simulink model "HANcoder_E407_GTSync_v3"  (R2018b)
settings: Solver=FixedStepDiscrete  StartTime=0.0  StopTime=1  FixedStep=0.01  RelTol=1e-3
PreLoadFcn:
  | librarySetup
  | eval([bdroot,'_startup']) %Calling [modelName]_startup.m
values from neighbouring files (symbols this model uses):
  frequency_IRQ = 100    [HANcoder_E407_GTSync_startup.m]    (also in HANcoder_E407_GTSync_v3_clean_startup.m = 99; HANcoder_E407_GTSync_v3_startup.m = 99)
  HANtuneOverride = Simulink.Parameter    [HANcoder_E407_GTSync_startup.m]    (also in HANcoder_E407_GTSync_v3_clean_startup.m; HANcoder_E407_GTSync_v3_startup.m)
  LED_ticks_toggle = 10000    [HANcoder_E407_GTSync_startup.m]    (also in HANcoder_E407_GTSync_v3_clean_startup.m; HANcoder_E407_GTSync_v3_startup.m)
  Master_Role = 1    [HANcoder_E407_GTSync_v3_clean_startup.m]    (also in HANcoder_E407_GTSync_v3_startup.m)
  matrix_rows = 2    [HANcoder_E407_GTSync_v3_clean_startup.m]    (also in HANcoder_E407_GTSync_v3_startup.m)
  Sync_ID = 1    [HANcoder_E407_GTSync_v3_clean_startup.m]    (also in HANcoder_E407_GTSync_v3_startup.m)
  time_difference_threshold = 500    [HANcoder_E407_GTSync_v3_clean_startup.m]    (also in HANcoder_E407_GTSync_v3_startup.m = 100)
  TM0 = 100    [HANcoder_E407_GTSync_v3_clean_startup.m]    (also in HANcoder_E407_GTSync_v3_startup.m = 0)
  TM1 = 20000    [HANcoder_E407_GTSync_v3_clean_startup.m]    (also in HANcoder_E407_GTSync_v3_startup.m = 25000)
  TM2 = 30000    [HANcoder_E407_GTSync_v3_clean_startup.m]    (also in HANcoder_E407_GTSync_v3_startup.m = 37500)
  TM3 = 40000    [HANcoder_E407_GTSync_v3_clean_startup.m]    (also in HANcoder_E407_GTSync_v3_startup.m)
  Vote1_ID = 12    [HANcoder_E407_GTSync_v3_clean_startup.m]    (also in HANcoder_E407_GTSync_v3_startup.m)
  Vote2_ID = 22    [HANcoder_E407_GTSync_v3_clean_startup.m]    (also in HANcoder_E407_GTSync_v3_startup.m)
  Vote3_ID = 32    [HANcoder_E407_GTSync_v3_clean_startup.m]    (also in HANcoder_E407_GTSync_v3_startup.m)
undefined symbols (not defined in the file or in its folder): votes
libraries: HANcoder_STM32_Target x20, simulink x3, simulink_extras x1
(part 1 of 2)
CloseFcn:
  | rtwprivate ssgencode ModelCloseRequest mytest
settings Model: Creator=Jason van Kolfschoten  LastModifiedBy=jordy
settings SolverCC: PositivePriorityOrder=on
settings DataIOCC: LimitDataPoints=on  SaveFormat=Array  SignalLoggingSaveFormat=ModelDataLogs  SaveOutput=off  SaveTime=off
settings OptimizationCC: BlockReduction=off  DefaultParameterBehavior=Inlined  InlineInvariantSignals=on  ExpressionDepthLimit=2147483647  StateBitsets=on  DataBitsets=on  ZeroExternalMemoryAtStartup=off  ZeroInternalMemoryAtStartup=off  InitFltsAndDblsToZero=on  NoFixptDivByZeroProtection=on  EfficientFloat2IntCast=on  LifeSpan=inf
settings DebuggingCC: SaveWithDisabledLinksMsg=none  SaveWithParameterizedLinksMsg=none  CheckSSInitialOutputMsg=off  UnderspecifiedInitializationDetection=Classic  MergeDetectMultiDrivingBlocksExec=none  SignalResolutionControl=TryResolveAll  SolverPrmCheckMsg=warning  InheritedTsInSrcMsg=none  MultiTaskDSMMsg=warning  MultiTaskCondExecSysMsg=none  ParameterPrecisionLossMsg=none  FcnCallInpInsideContextMsg=warning  StateNameClashWarn=warning  SFUnexpectedBacktrackingDiag=warning  SFNoUnconditionalDefaultTransitionDiag=warning  SFExecutionAtInitializationDiag=none
settings HardwareCC: ProdBitPerPointer=32  ProdBitPerSizeT=32  ProdBitPerPtrDiffT=32  ProdLargestAtomicFloat=None  ProdIntDivRoundTo=Undefined  ProdWordSize=32  ProdHWDeviceType=Generic->32-bit Embedded Processor  TargetEndianess=LittleEndian  TargetHWDeviceType=Infineon->TriCore
settings ModelReferenceCC: PropagateSignalLabelsOutOfModel=off
settings SFSimCC: SimUseLocalCustomCode=off  MATLABDynamicMemAlloc=off
settings RTWCC: SystemTargetFile=ert.tlc  MakeCommand=make_rtw SHELL= HANcoder_PORTABLE=1 HANcoder_BOOTLOADER=1  TemplateMakefile=STM32_E407_gcc.tmf  Description=Real-Time Workshop Embedded Coder (no auto configuration)  RTWUseLocalCustomCode=off
settings CodeAppCC: ForceParamTrailComments=on  IgnoreCustomStorageClasses=off  SimulinkDataObjDesc=on  CustomSymbolStrGlobalVar=rt$N$M  CustomSymbolStrType=$N$M  CustomSymbolStrFcn=$N$M$F  CustomSymbolStrMacro=$N$M  InsertBlockDesc=on  StateflowObjectComments=on  InternalIdentifier=Classic
settings ERTTargetCC: TargetFcnLib=ansi_tfl_tmw.mat  MultiwordLength=2048  IncludeMdlTerminateFcn=off  SuppressErrorStatus=on  SupportNonFinite=off  GenerateASAP2=on  InlinedParameterPlacement=NonHierarchical  ERTCustomFileTemplate=example_file_process.tlc  ConvertIfToSwitch=off  SuppressUnreachableDefaultCases=off
settings ConfigComp: CovMetricSettings=dw  CovHtmlReporting=on  CovSaveCumulativeToWorkspaceVar=on  CovSaveSingleToWorkspaceVar=on  CovExternalEMLEnable=off  DVMaxProcessTime=600  DVDisplayUnsatisfiableObjectives=on  DVAutomaticStubbing=off  DVModelCoverageObjectives=MCDC  DVMaxTestCaseSteps=500  DVTestSuiteOptimization=CombinedObjectives  DVDetectActiveLogic=on  DVSaveHarnessModel=on

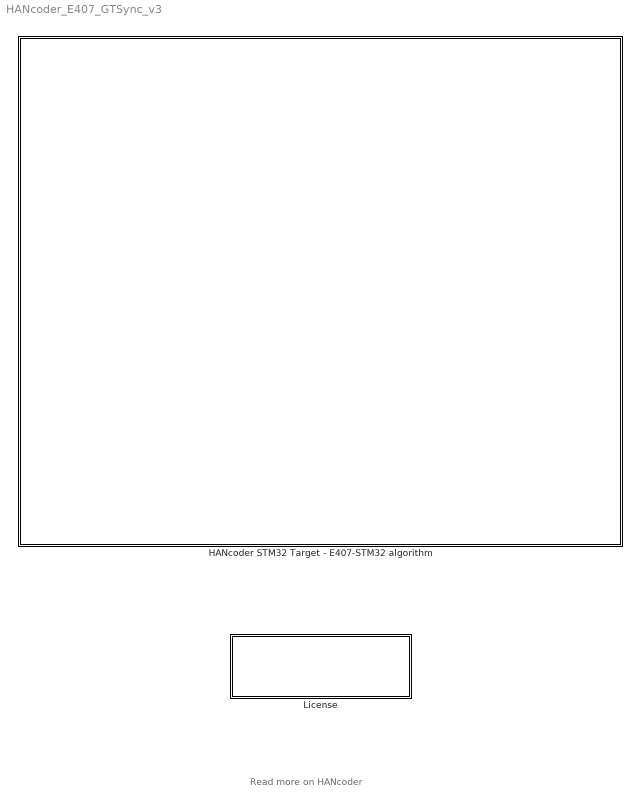
== system HANcoder_E407_GTSync_v3 ==
  note: Read more on HANcoder
  HANcoder STM32 Target - E407-STM32 algorithm : Subsystem  mask(TopLevelSubsystem){}
      settings: CopyFcn=HANcoderChecks('Copy');  NameChangeFcn=HANcoderChecks('NameChangeE407');  MoveFcn=HANcoderChecks('MoveE407');
      mask Display: image(imread('STM32_E407_HAN.jpg'))
  License : Subsystem  mask(License){}
      settings: NameChangeFcn=HANcoderChecks('NameChangeLicenseBlock');  OpenFcn=winopen('License.pdf')  MoveFcn=HANcoderChecks('MoveLicenseBlock');
      mask Display: disp(['End-User License Agreement\n','please read before use']);

== system HANcoder_E407_GTSync_v3/HANcoder STM32 Target - E407-STM32 algorithm ==
  note: Template model
  note: Global Variables
  Algorithm : Subsystem
  Base Sample Time config : HANcoder_STM32_Target/STM32-E407/System Config/Base Sample Time config  Tag=HANcoder_TARGET_STM32_E407  Description=HANcoder Target STM32-E407 blockset version 0.5  baseSampleTime=10  extraStack=0
      settings: SourceProductName=HANcoder STM32 Target
  Build settings : HANcoder_STM32_Target/STM32-E407/System Config/Build settings  Tag=HANcoder_TARGET_STM32_E407  AutoASAP2add=on  AutoFlash=USB
      settings: SourceProductName=HANcoder STM32 Target
  CAN config : HANcoder_STM32_Target/STM32-E407/System Config/CAN config  Tag=HANcoder_TARGET_STM32_E407  txBufSize=64  evBufSize=8  canBus1=off  baudRate1=500  rxMask1=hex2dec('00000000')  rxCode1=hex2dec('00000000')  rxMode1=Receive only 11-bit message identifiers  canBus2=on  baudRate2=500  rxMask2=hex2dec('00000000')  rxCode2=hex2dec('00000000')  rxMode2=Receive only 11-bit message identifiers
      settings: SourceProductName=HANcoder STM32 Target
  Custom ID config : HANcoder_STM32_Target/STM32-E407/System Config/Custom ID config  Tag=HANcoder_TARGET_STM32_E407  softID=softwareID  softNUM=1
      settings: SourceProductName=HANcoder STM32 Target
  Data Store Memory2 : DataStoreMemory  DataStoreName=local_ticks_mem_IRQ  ReadBeforeWriteMsg=warning  WriteAfterWriteMsg=warning  WriteAfterReadMsg=warning  ShowAdditionalParam=off  OutDataTypeStr=uint32
  Global Ticks Increment : Subsystem
  Inputs : Subsystem
  Operation Mode : Subsystem
  Outputs : Subsystem
  System information : Subsystem
  XCP on CAN config : HANcoder_STM32_Target/STM32-E407/System Config/XCP on CAN config  Tag=HANcoder_TARGET_STM32_E407  canBus=CAN 2  croID=hex2dec('665')  dtoID=hex2dec('666')
      settings: SourceProductName=HANcoder STM32 Target
  XCP on USB config : HANcoder_STM32_Target/STM32-E407/System Config/XCP on USB config  Tag=HANcoder_TARGET_STM32_E407
      settings: SourceProductName=HANcoder STM32 Target
  wires:
  Operation Mode/1(Clock_State) -> Global Ticks Increment/1(Clock_State)
  Inputs/1(Button) -> Operation Mode/1(Button_State), Algorithm/1(Button)

== system HANcoder_E407_GTSync_v3/License ==

== system HANcoder_E407_GTSync_v3/HANcoder STM32 Target - E407-STM32 algorithm/Algorithm ==
  note: The button or the HANtuneOverride parameter
      | switches between the two frequencies.
  note: Here the algorithm can be placed. No hardware dependent blocks should be used here.
  note: Switch LED frequency when button is pressed
  Button : Inport
  10Hz Counter Limiter : simulink/Sources/Counter Limited  uplimit=1  tsamp=0.1
  5Hz Counter Limited : simulink/Sources/Counter Limited  uplimit=1  tsamp=0.2
  Constant : Constant  Value=HANtuneOverride  OutDataTypeStr=boolean
  Data Type Conversion : DataTypeConversion  OutDataTypeStr=boolean
  Logical Operator : Logic  Operator=OR  AllPortsSameDT=off  OutDataTypeStr=boolean
  Switch : Switch  Criteria=u2 > Threshold
  Terminator : Terminator
  wires:
  Data Type Conversion/1 -> Terminator/1  "LedValue"
  5Hz Counter Limited/1 -> Switch/3
  Switch/1 -> Data Type Conversion/1
  Button/1 -> Logical Operator/2
  Logical Operator/1 -> Switch/2
  Constant/1 -> Logical Operator/1
  10Hz Counter Limiter/1 -> Switch/1

== system HANcoder_E407_GTSync_v3/HANcoder STM32 Target - E407-STM32 algorithm/Global Ticks Increment ==
  Clock_State : Inport
  CAN Management : Subsystem
  Compare Event IRQ : HANcoder_STM32_Target/STM32-E407/Timer Outputs/Compare Event IRQ  Tag=HANcoder_TARGET_STM32_E407  pin=TIM4 - CON PD - 15 - 5V Tolerant
      settings: SourceProductName=HANcoder STM32 Target
  Constant1 : Constant  Value=frequency_IRQ - 1  OutDataTypeStr=uint16
  Constant2 : Constant  Value=3  OutDataTypeStr=uint8
  Data Store Memory2 : DataStoreMemory  DataStoreName=message_buffer  ReadBeforeWriteMsg=warning  WriteAfterWriteMsg=warning  WriteAfterReadMsg=warning  ShowAdditionalParam=off  OutDataTypeStr=uint32
  Digital Clock : DigitalClock  SampleTime=0.01
  Function-Call Subsystem : Subsystem  TreatAsAtomicUnit=on
  Output Compare Init1 : Subsystem  Tag=HANcoder_TARGET_STM32_E407  AncestorBlock=HANcoder_STM32_Target/STM32-E407/Timer Outputs/Output Compare Init  mask(Output Compare Init){moduleID=TIM4 - CON PD - 15 & 16 &n/a & n/a, frequency=1000000, enableIRQoutput=off}
      mask prompts: moduleID "Timer module"; frequency "Frequency (free running counter) [Hz]"; enableIRQoutput "Enable IRQ output"
      mask help:
      | Function
      | ========
      | Initializes the timer module to allow output compare functionality on the
      | module's channels.
      |
      | Parameters
      | ==========
      | Timer Module:
      |   Selects the timer module.
      |
      | Frequency:
      |   Frequency at which the 16-bit free running counter counts.
      |
      | Enable IRQ output
      |   Controls whether or not the IRQ output is available.
      |
      | Outport
      | =======
      | IRQ
      |   Allows connection of a function call subsystem for the free running
      |   counter overflow event.
      mask init:
      | moduleIDInfoStr = sfcn_timeout_init_mcb(2, moduleID, frequency, enableIRQoutput);
      settings: CopyFcn=sfcn_timeout_init_chk();  MoveFcn=drawLogos
      mask Help: web('sfcn_timeout_init.html');
      mask TypeOptions moduleID: TIM1 - CON PE - 12 & 14 & 16 & 17 | TIM2 - CON4 - D13 & n/a & n/a & n/a | TIM3 - CON4 - D12 & D11 & n/a & n/a | TIM4 - CON PD - 15 & 16 &n/a & n/a | TIM8 - UEXT - 3 & 4 & n/a & n/a | TIM9 - CON3 - D4 & D5 or PE - 8 & 9 | TIM10 - CON2 - A1 or CON PF - 9 | TIM11 - CON2 - A2 or CON PF - 10 | TIM13 - CON2 - A3 or CON PF - 11 | TIM14 - CON2 - A4 or CON PF - 12
      mask Callback moduleID: sfcn_timeout_init_chk();
      mask Display: fprintf('Output Compare Init\n%s', moduleIDInfoStr);patch([135 141 141],[8 14 2],[1 0 0]);patch([143 143 149],[14 2 8],[0 0 0.35]);
  Schedule Compare Event1 : HANcoder_STM32_Target/STM32-E407/Timer Outputs/Schedule Compare Event  Tag=HANcoder_TARGET_STM32_E407  pin=TIM4 - CON PD - 15 - 5V Tolerant  tsamp=-1
      settings: SourceProductName=HANcoder STM32 Target
  Send : Subsystem
  Terminator : Terminator
  wires:
  Clock_State/1 -> Function-Call Subsystem/1(Clock_State)
  Digital Clock/1 -> Terminator/1  "simulation_time"
  Constant2/1 -> Schedule Compare Event1/2
  Constant1/1 -> Schedule Compare Event1/1
  Compare Event IRQ/1 -> Function-Call Subsystem/Trigger
  CAN Management/1(Send New Msg) -> Send/Trigger
  Function-Call Subsystem/1(activate_CAN_management) -> CAN Management/Trigger

== system HANcoder_E407_GTSync_v3/HANcoder STM32 Target - E407-STM32 algorithm/Inputs ==
  note: The inputs and outputs are kept in a separate subsystem, this way the algorithm can easily be transferred to different hardware
  Digital Input : HANcoder_STM32_Target/STM32-E407/Digital Inputs/Digital Input  Tag=HANcoder_TARGET_STM32_E407  pinID=WKUP button  config=Pulldown  tsamp=-1
      settings: SourceProductName=HANcoder STM32 Target
  Button : Outport
  wires:
  Digital Input/1 -> Button/1

== system HANcoder_E407_GTSync_v3/HANcoder STM32 Target - E407-STM32 algorithm/Operation Mode ==
  note: Operation Mode
      | There are two modes of operation:
      | ( 0 ) Idle (Clock Off)
      | ( 1 ) Counting (Clock On)
      | In order to switch from one to the other the Olimexino button
      | must be pressed once. In this subsystem, with every negative
      | edge of the Button State, the Operation Mode will change from
      | one to the other.
  Button_State : Inport
  Constant : Constant  OutDataTypeStr=boolean
  Flip Flop T : Subsystem
  Clock_State : Outport
  wires:
  Constant/1 -> Flip Flop T/1(T)
  Button_State/1 -> Flip Flop T/2(Clk)
  Flip Flop T/1(Q) -> Clock_State/1

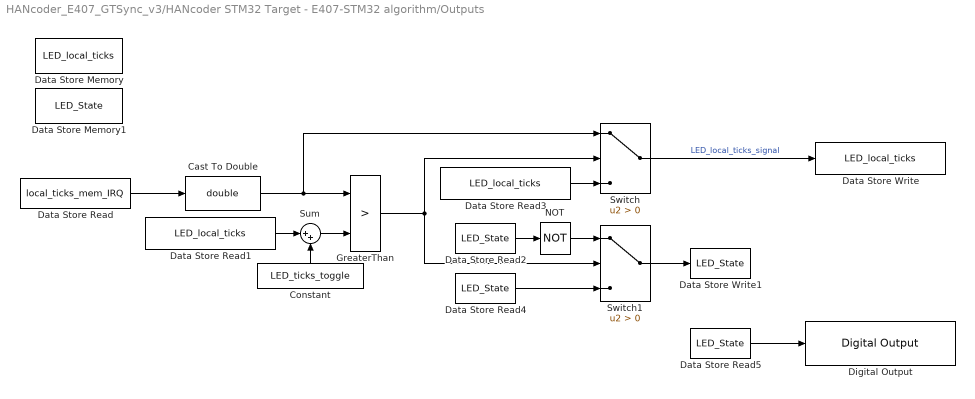
== system HANcoder_E407_GTSync_v3/HANcoder STM32 Target - E407-STM32 algorithm/Outputs ==
  Cast To Double : DataTypeConversion  OutDataTypeStr=double
  Constant : Constant  Value=LED_ticks_toggle
  Data Store Memory : DataStoreMemory  DataStoreName=LED_local_ticks  ReadBeforeWriteMsg=warning  WriteAfterWriteMsg=warning  WriteAfterReadMsg=warning  ShowAdditionalParam=off
  Data Store Memory1 : DataStoreMemory  DataStoreName=LED_State  ReadBeforeWriteMsg=warning  WriteAfterWriteMsg=warning  WriteAfterReadMsg=warning  ShowAdditionalParam=off  OutDataTypeStr=boolean
  Data Store Read : DataStoreRead  DataStoreName=local_ticks_mem_IRQ
  Data Store Read1 : DataStoreRead  DataStoreName=LED_local_ticks
  Data Store Read2 : DataStoreRead  DataStoreName=LED_State
  Data Store Read3 : DataStoreRead  DataStoreName=LED_local_ticks
  Data Store Read4 : DataStoreRead  DataStoreName=LED_State
  Data Store Read5 : DataStoreRead  DataStoreName=LED_State
  Data Store Write : DataStoreWrite  DataStoreName=LED_local_ticks
  Data Store Write1 : DataStoreWrite  DataStoreName=LED_State
  Digital Output : HANcoder_STM32_Target/STM32-E407/Digital Outputs/Digital Output  Tag=HANcoder_TARGET_STM32_E407  pinID=LED  config=Push pull  tsamp=-1
      settings: SourceProductName=HANcoder STM32 Target
  GreaterThan : RelationalOperator  Operator=>  OutDataTypeStr=boolean  RndMeth=Simplest
  NOT : Logic  Operator=NOT  IconShape=distinctive  AllPortsSameDT=off  OutDataTypeStr=boolean
  Sum : Sum  Inputs=|++
  Switch : Switch  Criteria=u2 > Threshold
  Switch1 : Switch  Criteria=u2 > Threshold
  wires:
  Data Store Read1/1 -> Sum/1
  Sum/1 -> GreaterThan/2
  Constant/1 -> Sum/2
  GreaterThan/1 -> Switch/2, Switch1/2
  Switch/1 -> Data Store Write/1  "LED_local_ticks_signal"
  Data Store Read/1 -> Cast To Double/1
  Data Store Read3/1 -> Switch/3
  Cast To Double/1 -> GreaterThan/1, Switch/1
  Switch1/1 -> Data Store Write1/1
  Data Store Read2/1 -> NOT/1
  NOT/1 -> Switch1/1
  Data Store Read4/1 -> Switch1/3
  Data Store Read5/1 -> Digital Output/1

== system HANcoder_E407_GTSync_v3/HANcoder STM32 Target - E407-STM32 algorithm/System information ==
  note: These blocks check the free memory: stack and heap and the CPU load,
      | this way you can see whether your software demands too much of the microcontroller
  Get CPU load : HANcoder_STM32_Target/STM32-E407/System Management/Get CPU load  Tag=HANcoder_TARGET_STM32_E407  mode=Current CPU load  tsamp=-1
      settings: SourceProductName=HANcoder STM32 Target
  Get free Heap : HANcoder_STM32_Target/STM32-E407/System Management/Get free Heap  Tag=HANcoder_TARGET_STM32_E407  tsamp=-1
      settings: SourceProductName=HANcoder STM32 Target
  Get free Stack : HANcoder_STM32_Target/STM32-E407/System Management/Get free Stack  Tag=HANcoder_TARGET_STM32_E407  taskIdx=Application Control Task  tsamp=-1
      settings: SourceProductName=HANcoder STM32 Target
  Terminator : Terminator
  Terminator1 : Terminator
  Terminator2 : Terminator
  wires:
  Get CPU load/1 -> Terminator1/1  "SI_CPUload"
  Get free Stack/1 -> Terminator/1  "SI_FreeStack"
  Get free Heap/1 -> Terminator2/1  "SI_FreeHeap"

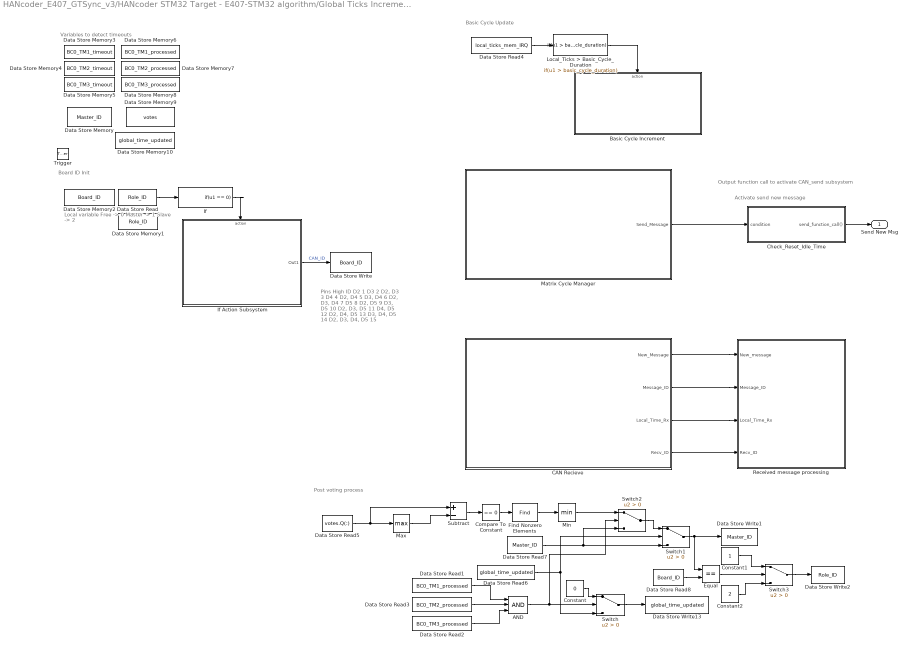
== system HANcoder_E407_GTSync_v3/HANcoder STM32 Target - E407-STM32 algorithm/Global Ticks Increment/CAN Management ==
  note: Post voting process
  note: Variables to detect timeouts
  note: Output function call to activate CAN_send subsystem
  note: Local variable
      |    Free     -> 0
      |    Master -> 1
      |    Slave   -> 2
  note: Pins High      		ID
      | D2                 		1
      | D3				2
      | D2, D3			3
      | D4				4
      | D2, D4			5
      | D3, D4			6
      | D2, D3, D4		7
      | D5				8
      | D2, D5			9
      | D3, D5			10
      | D2, D3, D5		11
      | D4, D5			12
      | D2, D4, D5		13
      | D3, D4, D5		14
      | D2, D3, D4, D5	15
  note: Board ID Init
  note: Activate send new message
  note: Basic Cycle Update
  Trigger : TriggerPort  TriggerType=function-call  VariantControl=Variant  PortDimensions=1
  AND : Logic  Inputs=3  IconShape=distinctive  AllPortsSameDT=off  OutDataTypeStr=boolean
  Basic Cycle Increment : Subsystem  TreatAsAtomicUnit=on
  CAN Recieve : Subsystem
  Check_Reset_Idle_Time : Stateflow chart  TreatAsAtomicUnit=on
  Compare To Constant : simulink/Logic and Bit Operations/Compare To Constant  relop===  const=0  OutDataTypeStr=boolean
  Constant : Constant  Value=0
  Constant1 : Constant
  Constant2 : Constant  Value=2
  Data Store Memory : DataStoreMemory  DataStoreName=Master_ID  ReadBeforeWriteMsg=warning  WriteAfterWriteMsg=warning  WriteAfterReadMsg=warning  InitialValue=1  ShowAdditionalParam=off
  Data Store Memory1 : DataStoreMemory  DataStoreName=Role_ID  ReadBeforeWriteMsg=warning  WriteAfterWriteMsg=warning  WriteAfterReadMsg=warning  ShowAdditionalParam=off
  Data Store Memory10 : DataStoreMemory  DataStoreName=global_time_updated  ReadBeforeWriteMsg=warning  WriteAfterWriteMsg=warning  WriteAfterReadMsg=warning  ShowAdditionalParam=off  OutDataTypeStr=boolean
  Data Store Memory2 : DataStoreMemory  DataStoreName=Board_ID  ReadBeforeWriteMsg=warning  WriteAfterWriteMsg=warning  WriteAfterReadMsg=warning  ShowAdditionalParam=off
  Data Store Memory3 : DataStoreMemory  DataStoreName=BC0_TM1_timeout  ReadBeforeWriteMsg=warning  WriteAfterWriteMsg=warning  WriteAfterReadMsg=warning  ShowAdditionalParam=off  OutDataTypeStr=boolean
  Data Store Memory4 : DataStoreMemory  DataStoreName=BC0_TM2_timeout  ReadBeforeWriteMsg=warning  WriteAfterWriteMsg=warning  WriteAfterReadMsg=warning  ShowAdditionalParam=off  OutDataTypeStr=boolean
  Data Store Memory5 : DataStoreMemory  DataStoreName=BC0_TM3_timeout  ReadBeforeWriteMsg=warning  WriteAfterWriteMsg=warning  WriteAfterReadMsg=warning  ShowAdditionalParam=off  OutDataTypeStr=boolean
  Data Store Memory6 : DataStoreMemory  DataStoreName=BC0_TM1_processed  ReadBeforeWriteMsg=warning  WriteAfterWriteMsg=warning  WriteAfterReadMsg=warning  ShowAdditionalParam=off  OutDataTypeStr=boolean
  Data Store Memory7 : DataStoreMemory  DataStoreName=BC0_TM2_processed  ReadBeforeWriteMsg=warning  WriteAfterWriteMsg=warning  WriteAfterReadMsg=warning  ShowAdditionalParam=off  OutDataTypeStr=boolean
  Data Store Memory8 : DataStoreMemory  DataStoreName=BC0_TM3_processed  ReadBeforeWriteMsg=warning  WriteAfterWriteMsg=warning  WriteAfterReadMsg=warning  ShowAdditionalParam=off  OutDataTypeStr=boolean
  Data Store Memory9 : DataStoreMemory  DataStoreName=votes  ReadBeforeWriteMsg=warning  WriteAfterWriteMsg=warning  WriteAfterReadMsg=warning  ShowAdditionalParam=off  OutDataTypeStr=Bus: vote_array
  Data Store Read : DataStoreRead  DataStoreName=Role_ID
  Data Store Read1 : DataStoreRead  DataStoreName=BC0_TM1_processed
  Data Store Read2 : DataStoreRead  DataStoreName=BC0_TM3_processed
  Data Store Read3 : DataStoreRead  DataStoreName=BC0_TM2_processed
  Data Store Read4 : DataStoreRead  DataStoreName=local_ticks_mem_IRQ
  Data Store Read5 : DataStoreRead  DataStoreName=votes  DataStoreElements=votes.Q(:)
  Data Store Read6 : DataStoreRead  DataStoreName=global_time_updated
  Data Store Read7 : DataStoreRead  DataStoreName=Master_ID
  Data Store Read8 : DataStoreRead  DataStoreName=Board_ID
  Data Store Write : DataStoreWrite  DataStoreName=Board_ID
  Data Store Write1 : DataStoreWrite  DataStoreName=Master_ID
  Data Store Write13 : DataStoreWrite  DataStoreName=global_time_updated
  Data Store Write2 : DataStoreWrite  DataStoreName=Role_ID
  Equal : RelationalOperator  Operator===  OutDataTypeStr=boolean  RndMeth=Simplest
  Find Nonzero Elements : Find  NumberOfInputDimensions=3  IndexMode=Zero-based
  If : If  IfExpression=u1 == 0  ShowElse=off
  If Action Subsystem : Subsystem  TreatAsAtomicUnit=on
  Local_Ticks > Basic_Cycle_Duration : If  IfExpression=u1 > basic_cycle_duration  ShowElse=off
  Matrix Cycle Manager : Subsystem
  Max : MinMax  Function=max
  Min : MinMax
  Received message processing : Subsystem  TreatAsAtomicUnit=on
  Subtract : Sum  Inputs=+-
  Switch{,1..3} (4 alike) : Switch  Criteria=u2 > Threshold
  Send New Msg : Outport
  wires:
  If/1 -> If Action Subsystem/Action
  If Action Subsystem/1(Out1) -> Data Store Write/1  "CAN_ID"
  Data Store Read/1 -> If/1
  Matrix Cycle Manager/1(Send_Message) -> Check_Reset_Idle_Time/1(condition)
  Check_Reset_Idle_Time/1(send_function_call()) -> Send New Msg/1
  CAN Recieve/1(New_Message) -> Received message processing/1(New_message)
  CAN Recieve/2(Message_ID) -> Received message processing/2(Message_ID)
  CAN Recieve/3(Local_Time_Rx) -> Received message processing/3(Local_Time_Rx)
  Data Store Read4/1 -> Local_Ticks > Basic_Cycle_Duration/1
  Local_Ticks > Basic_Cycle_Duration/1 -> Basic Cycle Increment/Action
  CAN Recieve/4(Recv_ID) -> Received message processing/4(Recv_ID)
  Data Store Read1/1 -> AND/1
  Data Store Read2/1 -> AND/3
  Data Store Read3/1 -> AND/2
  Data Store Read5/1 -> Max/1, Subtract/1
  Subtract/1 -> Compare To Constant/1
  Compare To Constant/1 -> Find Nonzero Elements/1
  Find Nonzero Elements/1 -> Min/1
  Max/1 -> Subtract/2
  Switch/1 -> Data Store Write13/1
  Constant/1 -> Switch/1
  AND/1 -> Switch2/2, Switch/2
  Data Store Read7/1 -> Switch1/3, Switch2/3
  Min/1 -> Switch2/1
  Switch1/1 -> Equal/1, Data Store Write1/1
  Data Store Read6/1 -> Switch1/2, Switch/3
  Switch2/1 -> Switch1/1
  Equal/1 -> Switch3/2
  Data Store Read8/1 -> Equal/2
  Switch3/1 -> Data Store Write2/1
  Constant1/1 -> Switch3/1
  Constant2/1 -> Switch3/3

== system HANcoder_E407_GTSync_v3/HANcoder STM32 Target - E407-STM32 algorithm/Global Ticks Increment/Function-Call Subsystem ==
  note: Counter Reset
  note: Tick Counter Increment
  Clock_State : Inport
  function : TriggerPort  TriggerType=function-call  VariantControl=Variant
  Check_Reset_Idle_Time : Stateflow chart  TreatAsAtomicUnit=on
  Constant : Constant  OutDataTypeStr=uint32
  Data Store Read : DataStoreRead  DataStoreName=local_ticks_mem_IRQ
  Data Store Read1 : DataStoreRead  DataStoreName=local_ticks_mem_IRQ
  Data Store Write : DataStoreWrite  DataStoreName=local_ticks_mem_IRQ
  Even_Tick : Stateflow chart  TreatAsAtomicUnit=on
  Odd_Tick : Stateflow chart  TreatAsAtomicUnit=on
  Reset Free Running Counter1 : HANcoder_STM32_Target/STM32-E407/Timer Outputs/Reset Free Running Counter  Tag=HANcoder_TARGET_STM32_E407  moduleID=TIM4 - CON PD - 15 & 16 &n/a & n/a
      settings: SourceProductName=HANcoder STM32 Target
  Reset Free Running Counter2 : HANcoder_STM32_Target/STM32-E407/Timer Outputs/Reset Free Running Counter  Tag=HANcoder_TARGET_STM32_E407  moduleID=TIM4 - CON PD - 15 & 16 &n/a & n/a
      settings: SourceProductName=HANcoder STM32 Target
  Sum : Sum
  Switch : Switch  Criteria=u2 > Threshold
  activate_CAN_management : Outport
  wires:
  Constant/1 -> Sum/2
  Switch/1 -> Data Store Write/1, Even_Tick/1(current_tick), Odd_Tick/1(current_tick)  "local_ticks_interrupt"
  Clock_State/1 -> Switch/2, Check_Reset_Idle_Time/1(WKUP_state)
  Data Store Read/1 -> Sum/1
  Sum/1 -> Switch/1
  Data Store Read1/1 -> Switch/3
  Even_Tick/1(rise_edge_at_even) -> Reset Free Running Counter1/Trigger  "even"
  Odd_Tick/1(rise_edge_at_odd) -> Reset Free Running Counter2/Trigger  "odd"
  Check_Reset_Idle_Time/1(WKUP_CAN()) -> activate_CAN_management/1

== system HANcoder_E407_GTSync_v3/HANcoder STM32 Target - E407-STM32 algorithm/Global Ticks Increment/Output Compare Init1 ==
  S-Function : S-Function  FunctionName=sfcn_timeout_init  SFunctionDeploymentMode=off  EnableBusSupport=off
  Term1 : Terminator
  wires:
  S-Function/1 -> Term1/1

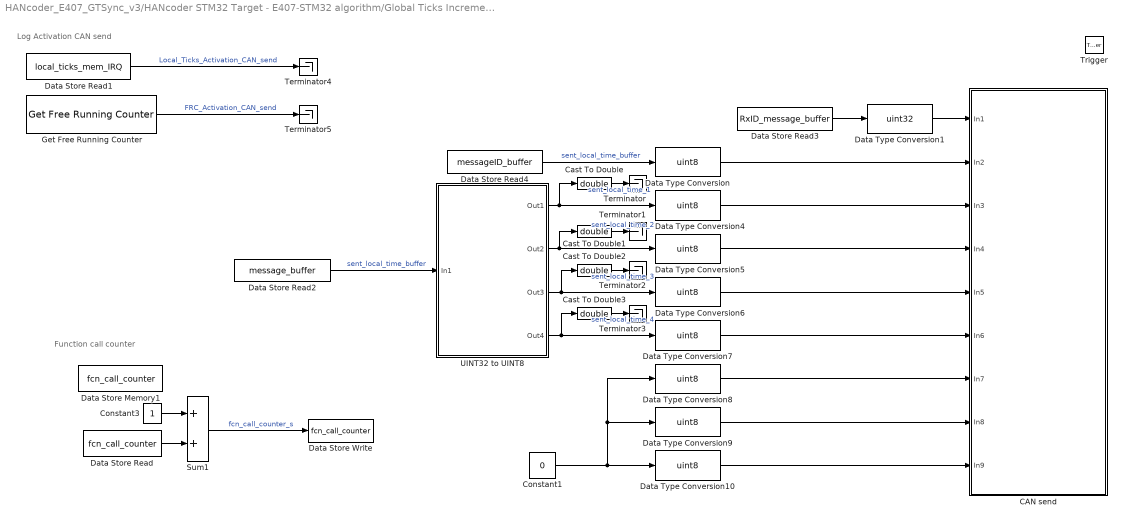
== system HANcoder_E407_GTSync_v3/HANcoder STM32 Target - E407-STM32 algorithm/Global Ticks Increment/Send ==
  note: Log Activation CAN send
  note: Function call counter
  Trigger : TriggerPort  TriggerType=function-call  VariantControl=Variant  PortDimensions=1
  CAN send : Subsystem  Tag=HANcoder_TARGET_STM32_E407  AncestorBlock=HANcoder_STM32_Target/STM32-E407/CAN/CAN/CAN send  mask(CAN send){canBus=CAN 2, frameType=Standard (11 bit), inputNumber=8, dataType=uint8, byteOrder=off, tsamp=-1}
      mask prompts: canBus "CAN channel"; frameType "Identifier type"; inputNumber "Input ports"; dataType "Input datatype"; byteOrder "Byte order: Checked = MSB first, unchecked = LSB first."; tsamp "Sample time"
      mask help:
      | Function
      | ==========
      | Send a message on the CAN channel.
      |
      | Parameters
      | ==========
      | CAN channel:           The CAN channel to send the message on.
      | Identifier type:         normal or extended ID's
      | Input ports:              The amount of input ports
      | Input datatype:        The datatype of the input ports
      | Byte order:               Select MSB or LSB first
      | Sample time:            -1 or divisible by base sample time [seconds]
      |
      | Input
      | ==========
      | Port 1:                   CAN ID(uint32) in hexadecimal ie: hex2dec('0a')
      | Port 2..9                CAN message data
      mask init:
      | sfcn_can_send_mcb(canBus, frameType, inputNumber, dataType, byteOrder)
      settings: MoveFcn=drawLogos
      mask Help: web('sfcn_can_send.html');
      mask TypeOptions canBus: CAN 1 | CAN 2
      mask TypeOptions frameType: Standard (11 bit) | Extended (29 bit)
      mask TypeOptions dataType: int8 | uint8 | int16 | uint16 | int32 | uint32 | boolean
      mask Display:
      | fprintf('Send on\nCAN %x', canBus);
      | port_label('input', 1, 'ID');patch([140 146 146],[8 14 2],[1 0 0]);patch([148 148 154],[14 2 8],[0 0 0.35]);
  Cast To Double{,1..3} (4 alike) : DataTypeConversion  OutDataTypeStr=double
  Constant1 : Constant  Value=0
  Constant3 : Constant  OutDataTypeStr=uint32
  Data Store Memory1 : DataStoreMemory  DataStoreName=fcn_call_counter  ReadBeforeWriteMsg=warning  WriteAfterWriteMsg=warning  WriteAfterReadMsg=warning  ShowAdditionalParam=off  OutDataTypeStr=uint32
  Data Store Read : DataStoreRead  DataStoreName=fcn_call_counter
  Data Store Read1 : DataStoreRead  DataStoreName=local_ticks_mem_IRQ
  Data Store Read2 : DataStoreRead  DataStoreName=message_buffer
  Data Store Read3 : DataStoreRead  DataStoreName=RxID_message_buffer
  Data Store Read4 : DataStoreRead  DataStoreName=messageID_buffer
  Data Store Write : DataStoreWrite  DataStoreName=fcn_call_counter
  Data Type Conversion{,4..10} (8 alike) : DataTypeConversion  OutDataTypeStr=uint8
  Data Type Conversion1 : DataTypeConversion  OutDataTypeStr=uint32
  Get Free Running Counter : HANcoder_STM32_Target/STM32-E407/Timer Outputs/Get Free Running Counter  Tag=HANcoder_TARGET_STM32_E407  moduleID=TIM4 - CON PD - 15 & 16 &n/a & n/a  tsamp=-1
      settings: SourceProductName=HANcoder STM32 Target
  Sum1 : Sum
  Terminator{,1..5} (6 alike) : Terminator
  UINT32 to UINT8 : Subsystem
  wires:
  Data Type Conversion10/1 -> CAN send/9(In9)
  Data Type Conversion/1 -> CAN send/2(In2)
  Data Type Conversion1/1 -> CAN send/1(In1)
  Data Type Conversion9/1 -> CAN send/8(In8)
  Data Type Conversion8/1 -> CAN send/7(In7)
  Data Store Read3/1 -> Data Type Conversion1/1
  Data Type Conversion5/1 -> CAN send/4(In4)
  Data Type Conversion4/1 -> CAN send/3(In3)
  Data Type Conversion6/1 -> CAN send/5(In5)
  Data Type Conversion7/1 -> CAN send/6(In6)
  Constant1/1 -> Data Type Conversion10/1, Data Type Conversion8/1, Data Type Conversion9/1
  UINT32 to UINT8/1(Out1) -> Cast To Double/1, Data Type Conversion4/1
  UINT32 to UINT8/2(Out2) -> Cast To Double1/1, Data Type Conversion5/1
  UINT32 to UINT8/3(Out3) -> Cast To Double2/1, Data Type Conversion6/1
  Cast To Double/1 -> Terminator/1  "sent_local_time_1"
  Cast To Double1/1 -> Terminator1/1  "sent_local_time_2"
  Cast To Double2/1 -> Terminator2/1  "sent_local_time_3"
  Cast To Double3/1 -> Terminator3/1  "sent_local_time_4"
  Data Store Read2/1 -> UINT32 to UINT8/1(In1)  "sent_local_time_buffer"
  Constant3/1 -> Sum1/1
  Data Store Read/1 -> Sum1/2
  Sum1/1 -> Data Store Write/1  "fcn_call_counter_s"
  Data Store Read1/1 -> Terminator4/1  "Local_Ticks_Activation_CAN_send"
  Get Free Running Counter/1 -> Terminator5/1  "FRC_Activation_CAN_send"
  UINT32 to UINT8/4(Out4) -> Data Type Conversion7/1, Cast To Double3/1
  Data Store Read4/1 -> Data Type Conversion/1  "sent_local_time_buffer"

== system HANcoder_E407_GTSync_v3/HANcoder STM32 Target - E407-STM32 algorithm/Operation Mode/Flip Flop T ==
  T : Inport  OutDataTypeStr=boolean
  Clk : Inport  Port=2  OutDataTypeStr=boolean
  J-K Flip-Flop : simulink_extras/Flip Flops/J-K Flip-Flop  initial_condition=0
      settings: SourceProductName=Simulink
  Terminator : Terminator
  Q : Outport  OutDataTypeStr=boolean
  wires:
  J-K Flip-Flop/2 -> Terminator/1
  T/1 -> J-K Flip-Flop/3, J-K Flip-Flop/1
  J-K Flip-Flop/1 -> Q/1
  Clk/1 -> J-K Flip-Flop/2

== system HANcoder_E407_GTSync_v3/HANcoder STM32 Target - E407-STM32 algorithm/Global Ticks Increment/CAN Management/Basic Cycle Increment ==
  note: Basic cycle counter
  Action Port : ActionPort  ActionType=then
  Add : Sum
  Constant : Constant  Value=matrix_rows
  Data Store Read4 : DataStoreRead  DataStoreName=basic_cycle_count
  Data Store Read5 : DataStoreRead  DataStoreName=basic_cycle_count
  Data Store Write3 : DataStoreWrite  DataStoreName=basic_cycle_count
  Increment : Constant  OutDataTypeStr=uint8
  LessThanOrEqual : RelationalOperator  Operator=<  OutDataTypeStr=boolean  RndMeth=Simplest
  Reset : Constant  Value=0  OutDataTypeStr=uint8
  Switch : Switch  Criteria=u2 > Threshold
  wires:
  Switch/1 -> Data Store Write3/1  "bc"
  Reset/1 -> Switch/3
  Data Store Read5/1 -> LessThanOrEqual/1
  Add/1 -> Switch/1
  Increment/1 -> Add/2
  Data Store Read4/1 -> Add/1
  LessThanOrEqual/1 -> Switch/2
  Constant/1 -> LessThanOrEqual/2

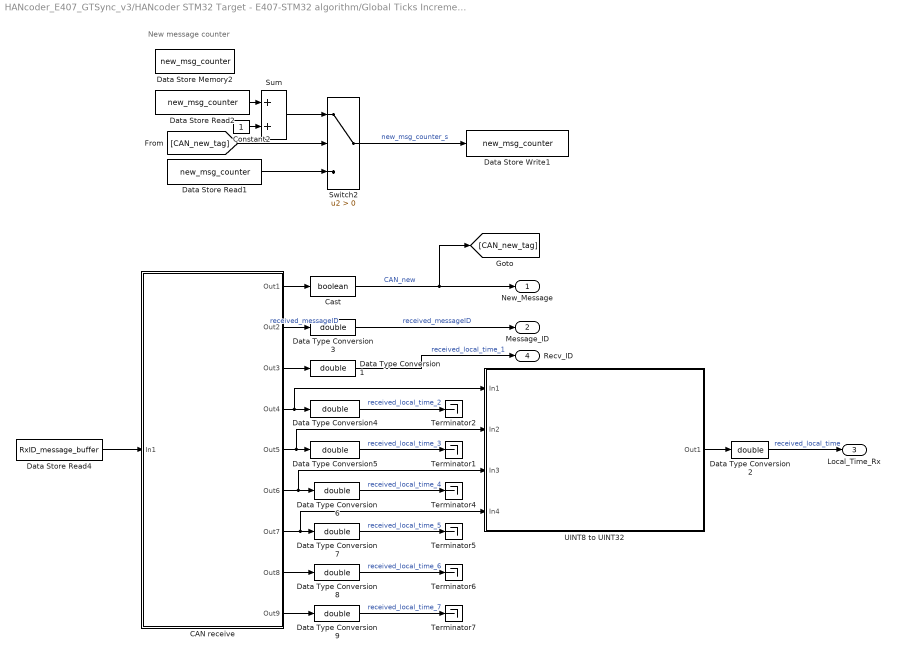
== system HANcoder_E407_GTSync_v3/HANcoder STM32 Target - E407-STM32 algorithm/Global Ticks Increment/CAN Management/CAN Recieve ==
  note: New message counter
  CAN receive : Subsystem  Tag=HANcoder_TARGET_STM32_E407  AncestorBlock=HANcoder_STM32_Target/STM32-E407/CAN/CAN/CAN receive  mask(CAN receive){canBus=CAN 2, outputNumber=8, dataType=uint8, byteOrder=off, tsamp=-1}
      mask prompts: canBus "CAN channel"; outputNumber "Output ports"; dataType "Output datatype"; byteOrder "Byte order: Checked = MSB first, unchecked = LSB first."; tsamp "Sample time"
      mask help:
      | Function
      | ==========
      | Receive the newest message from the specified CAN channel.
      |
      | Parameters
      | ==========
      | CAN channel:             The CAN channel to send the message on.
      | Output ports:             The amount of output ports
      | Output datatype:       The datatype of the output ports
      | Byte order:                 Select MSB or LSB first
      | Sample time:              -1 or divisible by base sample time [seconds]
      |
      | Input
      | ==========
      | Port 1:                       CAN ID(uint32) in hexadecimal ie: hex2dec('0a')
      |
      | Output
      | ==========
      | Port 1:                       Checks for new message(int8)
      | Port 2..9                     Message data
      mask init:
      | sfcn_can_receive_mcb(canBus, outputNumber, dataType, byteOrder)
      settings: MoveFcn=drawLogos
      mask Help: web('sfcn_can_receive.html');
      mask TypeOptions canBus: CAN 1 | CAN 2
      mask TypeOptions dataType: int8 | uint8 | int16 | uint16 | int32 | uint32 | boolean
      mask Display:
      | fprintf('Receive on\nCAN %x', canBus);
      | port_label('output', 1, 'new');
      | port_label('input', 1, 'ID');patch([155 161 161],[8 14 2],[1 0 0]);patch([163 163 169],[14 2 8],[0 0 0.35]);
  Cast : DataTypeConversion  OutDataTypeStr=boolean
  Constant2 : Constant  OutDataTypeStr=uint32
  Data Store Memory2 : DataStoreMemory  DataStoreName=new_msg_counter  ReadBeforeWriteMsg=warning  WriteAfterWriteMsg=warning  WriteAfterReadMsg=warning  ShowAdditionalParam=off  OutDataTypeStr=uint32
  Data Store Read1 : DataStoreRead  DataStoreName=new_msg_counter
  Data Store Read2 : DataStoreRead  DataStoreName=new_msg_counter
  Data Store Read4 : DataStoreRead  DataStoreName=RxID_message_buffer
  Data Store Write1 : DataStoreWrite  DataStoreName=new_msg_counter
  Data Type Conversion{1..9} (9 alike) : DataTypeConversion  OutDataTypeStr=double
  Sum : Sum
  Switch2 : Switch  Criteria=u2 > Threshold
  Terminator{1..2,4..7} (6 alike) : Terminator
  UINT8 to UINT32 : Subsystem
  New_Message : Outport
  Message_ID : Outport  Port=2
  Local_Time_Rx : Outport  Port=3
  Recv_ID : Outport  Port=4
  wires:
  CAN receive/9(Out9) -> Data Type Conversion9/1
  CAN receive/6(Out6) -> UINT8 to UINT32/3(In3), Data Type Conversion6/1
  Data Type Conversion7/1 -> Terminator5/1  "received_local_time_5"
  CAN receive/4(Out4) -> UINT8 to UINT32/1(In1), Data Type Conversion4/1
  CAN receive/8(Out8) -> Data Type Conversion8/1
  Data Type Conversion5/1 -> Terminator1/1  "received_local_time_3"
  CAN receive/1(Out1) -> Cast/1
  Data Type Conversion4/1 -> Terminator2/1  "received_local_time_2"
  Data Type Conversion1/1 -> Recv_ID/1  "received_local_time_1"
  CAN receive/3(Out3) -> Data Type Conversion1/1
  Data Type Conversion3/1 -> Message_ID/1  "received_messageID"
  Data Type Conversion8/1 -> Terminator6/1  "received_local_time_6"
  Data Type Conversion9/1 -> Terminator7/1  "received_local_time_7"
  CAN receive/5(Out5) -> UINT8 to UINT32/2(In2), Data Type Conversion5/1
  CAN receive/2(Out2) -> Data Type Conversion3/1  "received_messageID"
  CAN receive/7(Out7) -> UINT8 to UINT32/4(In4), Data Type Conversion7/1
  UINT8 to UINT32/1(Out1) -> Data Type Conversion2/1
  Cast/1 -> [CAN_new_tag], New_Message/1  "CAN_new"
  Data Store Read1/1 -> Switch2/3
  Constant2/1 -> Sum/2
  Sum/1 -> Switch2/1
  Switch2/1 -> Data Store Write1/1  "new_msg_counter_s"
  Data Store Read2/1 -> Sum/1
  Data Store Read4/1 -> CAN receive/1(In1)
  Data Type Conversion6/1 -> Terminator4/1  "received_local_time_4"
  [CAN_new_tag] -> Switch2/2
  Data Type Conversion2/1 -> Local_Time_Rx/1  "received_local_time"

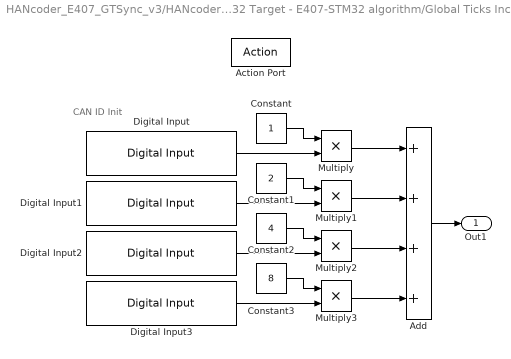
== system HANcoder_E407_GTSync_v3/HANcoder STM32 Target - E407-STM32 algorithm/Global Ticks Increment/CAN Management/If Action Subsystem ==
  note: CAN ID Init
  Action Port : ActionPort  ActionType=then
  Add : Sum  Inputs=++++
  Constant : Constant
  Constant1 : Constant  Value=2
  Constant2 : Constant  Value=4
  Constant3 : Constant  Value=8
  Digital Input : HANcoder_STM32_Target/STM32-E407/Digital Inputs/Digital Input  Tag=HANcoder_TARGET_STM32_E407  pinID=CON3 - D2 - 5V Tolerant  config=Pulldown  tsamp=-1
      settings: SourceProductName=HANcoder STM32 Target
  Digital Input1 : HANcoder_STM32_Target/STM32-E407/Digital Inputs/Digital Input  Tag=HANcoder_TARGET_STM32_E407  pinID=CON3 - D3 - 5V Tolerant  config=Pulldown  tsamp=-1
      settings: SourceProductName=HANcoder STM32 Target
  Digital Input2 : HANcoder_STM32_Target/STM32-E407/Digital Inputs/Digital Input  Tag=HANcoder_TARGET_STM32_E407  pinID=CON3 - D4 - 5V Tolerant  config=Pulldown  tsamp=-1
      settings: SourceProductName=HANcoder STM32 Target
  Digital Input3 : HANcoder_STM32_Target/STM32-E407/Digital Inputs/Digital Input  Tag=HANcoder_TARGET_STM32_E407  pinID=CON3 - D5 - 5V Tolerant  config=Pulldown  tsamp=-1
      settings: SourceProductName=HANcoder STM32 Target
  Multiply{,1..3} (4 alike) : Product
  Out1 : Outport
  wires:
  Constant1/1 -> Multiply1/1
  Add/1 -> Out1/1
  Constant3/1 -> Multiply3/1
  Constant2/1 -> Multiply2/1
  Multiply2/1 -> Add/3
  Digital Input3/1 -> Multiply3/2
  Digital Input1/1 -> Multiply1/2
  Multiply3/1 -> Add/4
  Multiply1/1 -> Add/2
  Digital Input2/1 -> Multiply2/2
  Multiply/1 -> Add/1
  Digital Input/1 -> Multiply/2
  Constant/1 -> Multiply/1

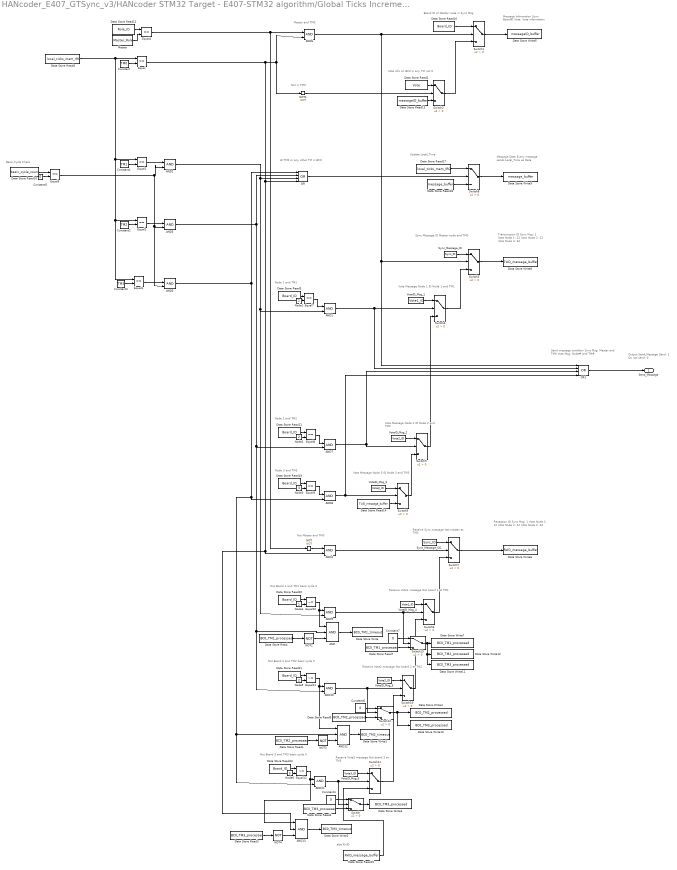
== system HANcoder_E407_GTSync_v3/HANcoder STM32 Target - E407-STM32 algorithm/Global Ticks Increment/CAN Management/Matrix Cycle Manager ==
  note: else RxID
  note: Receive Vote3 message
      | Not board 3 at TM3
  note: Receive Vote2 message
      | Not board 2 at TM2
  note: Receive Vote1 message
      | Not board 1 at TM1
  note: Not Board 3 and TM3
      | basic cycle 0
  note: Not Board 2 and TM2
      | basic cycle 0
  note: Not Board 1 and TM1
      | basic cycle 0
  note: Receive Sync message
      | Not master at TM0
  note: Reception ID
      |    Sync Msg: 1
      |    Vote Node 1: 12
      |    Vote Node 2: 22
      |    Vote Node 3: 32
  note: Vote Message Node 3 ID
      | Node 3 and TM3
  note: Node 3 and TM3
  note: Node 2 and TM2
  note: Vote Message Node 2 ID
      | Node 2 and TM2
  note: Output Send_Message
      | Send: 1
      | Do not send: 0
  note: Send message condition
      | Sync Msg: Master and TM0
      | Vote Msg: Node# and TM#
  note: Transmission ID
      |    Sync Msg: 1
      |    Vote Node 1: 12
      |    Vote Node 2: 22
      |    Vote Node 3: 32
  note: Vote Message Node 1 ID
      | Node 1 and TM1
  note: Node 1 and TM1
  note: Not Master and TM0
  note: Sync Message ID
      | Master node and TM0
  note: Message Data
      |    Every message sends
      |    Local_Time as Data
  note: Update Local_Time
  note: At TM0 or
      | any other TM in BC0
  note: Message Information
      |    Sync: BoardID
      |    Vote: Vote information
  note: Not in TM0
  note: Vote info on BC0 in any TM not 0
  note: Board ID of Master node in Sync Msg
  note: Master and TM0
  note: Basic Cycle Check
  AND : Logic  Inputs=3  IconShape=distinctive  AllPortsSameDT=off  OutDataTypeStr=boolean
  AND{1..11} (11 alike) : Logic  IconShape=distinctive  AllPortsSameDT=off  OutDataTypeStr=boolean
  AND12 : Logic  Inputs=3  IconShape=distinctive  AllPortsSameDT=off  OutDataTypeStr=boolean
  AND13 : Logic  Inputs=3  IconShape=distinctive  AllPortsSameDT=off  OutDataTypeStr=boolean
  Constant : Constant  Value=TM0
  Constant1 : Constant  Value=TM1
  Constant2 : Constant  Value=TM2
  Constant3 : Constant  Value=TM3
  Constant{4..7} (4 alike) : Constant  Value=0
  Data Store Read : DataStoreRead  DataStoreName=BC0_TM1_processed
  Data Store Read1 : DataStoreRead  DataStoreName=BC0_TM2_processed
  Data Store Read10 : DataStoreRead  DataStoreName=basic_cycle_count
  Data Store Read{5,11,16,19..21,23} (7 alike) : DataStoreRead  DataStoreName=Board_ID
  Data Store Read12 : DataStoreRead  DataStoreName=Role_ID
  Data Store Read13 : DataStoreRead  DataStoreName=messageID_buffer
  Data Store Read14 : DataStoreRead  DataStoreName=TxID_message_buffer
  Data Store Read15 : DataStoreRead  DataStoreName=RxID_message_buffer
  Data Store Read17 : DataStoreRead  DataStoreName=local_ticks_mem_IRQ
  Data Store Read18 : DataStoreRead  DataStoreName=message_buffer
  Data Store Read2 : DataStoreRead  DataStoreName=Vote
  Data Store Read3 : DataStoreRead  DataStoreName=BC0_TM3_processed
  Data Store Read4 : DataStoreRead  DataStoreName=BC0_TM3_processed
  Data Store Read6 : DataStoreRead  DataStoreName=BC0_TM2_processed
  Data Store Read7 : DataStoreRead  DataStoreName=BC0_TM1_processed
  Data Store Read9 : DataStoreRead  DataStoreName=local_ticks_mem_IRQ
  Data Store Write : DataStoreWrite  DataStoreName=BC0_TM1_timeout
  Data Store Write1 : DataStoreWrite  DataStoreName=BC0_TM2_timeout
  Data Store Write10 : DataStoreWrite  DataStoreName=BC0_TM3_processed
  Data Store Write11 : DataStoreWrite  DataStoreName=BC0_TM3_processed
  Data Store Write12 : DataStoreWrite  DataStoreName=BC0_TM2_processed
  Data Store Write2 : DataStoreWrite  DataStoreName=BC0_TM3_timeout
  Data Store Write3 : DataStoreWrite  DataStoreName=BC0_TM3_processed
  Data Store Write4 : DataStoreWrite  DataStoreName=BC0_TM2_processed
  Data Store Write5 : DataStoreWrite  DataStoreName=messageID_buffer
  Data Store Write6 : DataStoreWrite  DataStoreName=RxID_message_buffer
  Data Store Write7 : DataStoreWrite  DataStoreName=BC0_TM1_processed
  Data Store Write8 : DataStoreWrite  DataStoreName=TxID_message_buffer
  Data Store Write9 : DataStoreWrite  DataStoreName=message_buffer
  Equal{,1..5,7..9} (9 alike) : RelationalOperator  Operator===  OutDataTypeStr=boolean  RndMeth=Simplest
  Equal10 : RelationalOperator  Operator=~=  OutDataTypeStr=boolean  RndMeth=Simplest
  Equal11 : RelationalOperator  Operator=~=  OutDataTypeStr=boolean  RndMeth=Simplest
  Equal12 : RelationalOperator  Operator=~=  OutDataTypeStr=boolean  RndMeth=Simplest
  Master : Constant  Value=Master_Role
  NOT{,1..4} (5 alike) : Logic  Operator=NOT  IconShape=distinctive  AllPortsSameDT=off  OutDataTypeStr=boolean
  Node1 : Constant
  Node2 : Constant  Value=2
  Node3 : Constant  Value=3
  Node4 : Constant
  Node5 : Constant  Value=2
  Node6 : Constant  Value=3
  OR : Logic  Operator=OR  Inputs=4  IconShape=distinctive  AllPortsSameDT=off  OutDataTypeStr=boolean
  OR1 : Logic  Operator=OR  Inputs=4  IconShape=distinctive  AllPortsSameDT=off  OutDataTypeStr=boolean
  Switch{,1..13} (14 alike) : Switch  Criteria=u2 > Threshold
  Sync_Message_ID : Constant  Value=Sync_ID
  Sync_Message_ID1 : Constant  Value=Sync_ID
  VoteID_Msg_1 : Constant  Value=Vote1_ID
  VoteID_Msg_2 : Constant  Value=Vote2_ID
  VoteID_Msg_3 : Constant  Value=Vote3_ID
  VoteID_Msg_4 : Constant  Value=Vote1_ID
  VoteID_Msg_5 : Constant  Value=Vote2_ID
  VoteID_Msg_6 : Constant  Value=Vote3_ID
  Send_Message : Outport
  wires:
  Data Store Read9/1 -> Equal/1, Equal3/1, Equal2/1, Equal1/1
  Switch5/1 -> Switch4/3
  NOT1/1 -> Switch2/2
  Node4/1 -> Equal10/2
  VoteID_Msg_2/1 -> Switch5/1
  Data Store Read16/1 -> Switch1/1
  AND2/1 -> OR/3, AND1/2, AND9/2
  Data Store Read21/1 -> Equal11/1
  Constant3/1 -> Equal3/2
  OR/1 -> Switch8/2
  Switch8/1 -> Data Store Write9/1
  Switch3/1 -> Data Store Write8/1
  Node1/1 -> Equal7/2
  Equal10/1 -> AND/1, AND9/1
  Data Store Read2/1 -> Switch2/1
  Equal4/1 -> AND6/1, NOT/1
  Equal8/1 -> AND7/1
  Node5/1 -> Equal11/2
  Equal5/1 -> AND5/2, AND3/2, AND2/2
  Data Store Read10/1 -> Equal5/1
  Data Store Read20/1 -> Equal10/1
  Switch2/1 -> Switch1/3
  VoteID_Msg_1/1 -> Switch4/1
  Constant5/1 -> Equal5/2
  Constant/1 -> Equal/2
  VoteID_Msg_6/1 -> Switch11/1
  Data Store Read17/1 -> Switch8/1
  VoteID_Msg_3/1 -> Switch9/1
  Switch11/1 -> Switch10/3
  Data Store Read5/1 -> Equal7/1
  Constant2/1 -> Equal2/2
  Equal3/1 -> AND5/1
  Constant1/1 -> Equal1/2
  Data Store Read11/1 -> Equal8/1
  Switch9/1 -> Switch5/3
  AND3/1 -> OR/2, AND10/2, AND/2, AND7/2
  Node2/1 -> Equal8/2
  Sync_Message_ID1/1 -> Switch7/1
  Data Store Read23/1 -> Equal12/1
  VoteID_Msg_5/1 -> Switch10/1
  Data Store Read18/1 -> Switch8/3
  AND7/1 -> Switch5/2, OR1/3
  Switch10/1 -> Switch6/3
  VoteID_Msg_4/1 -> Switch6/1
  Equal1/1 -> AND2/1
  Equal2/1 -> AND3/1
  AND8/1 -> Switch9/2, OR1/4
  Switch6/1 -> Switch7/3
  Switch4/1 -> Switch3/3
  Data Store Read15/1 -> Switch11/3
  Data Store Read14/1 -> Switch9/3
  Sync_Message_ID/1 -> Switch3/1
  AND1/1 -> Switch4/2, OR1/2
  Switch7/1 -> Data Store Write6/1
  Node6/1 -> Equal12/2
  AND11/1 -> Switch/2, Switch11/2
  AND4/1 -> Switch7/2
  Equal9/1 -> AND8/1
  Data Store Read19/1 -> Equal9/1
  Node3/1 -> Equal9/2
  Switch1/1 -> Data Store Write5/1
  NOT/1 -> AND4/1
  AND6/1 -> Switch1/2, Switch3/2, OR1/1
  Equal7/1 -> AND1/1
  Data Store Read13/1 -> Switch2/3
  Master/1 -> Equal4/2
  Data Store Read12/1 -> Equal4/1
  OR1/1 -> Send_Message/1
  NOT2/1 -> AND/3
  Data Store Read/1 -> NOT2/1
  AND/1 -> Data Store Write/1
  Data Store Read1/1 -> NOT3/1
  Equal11/1 -> AND12/1, AND10/1
  AND12/1 -> Data Store Write1/1
  NOT3/1 -> AND12/3
  AND5/1 -> OR/1, AND11/2, AND12/2, AND8/2
  Data Store Read3/1 -> NOT4/1
  Equal12/1 -> AND13/1, AND11/1
  AND13/1 -> Data Store Write2/1
  NOT4/1 -> AND13/3
  Equal/1 -> AND6/2, NOT1/1, OR/4, AND13/2, AND4/2
  Switch/1 -> Data Store Write3/1
  Constant4/1 -> Switch/1
  Data Store Read4/1 -> Switch/3
  Constant6/1 -> Switch12/1
  AND10/1 -> Switch12/2, Switch10/2
  Switch12/1 -> Data Store Write10/1, Data Store Write4/1
  Data Store Read6/1 -> Switch12/3
  Constant7/1 -> Switch13/1
  AND9/1 -> Switch13/2, Switch6/2
  Switch13/1 -> Data Store Write11/1, Data Store Write12/1, Data Store Write7/1
  Data Store Read7/1 -> Switch13/3
